simulink model "model_3"  (R2021b)
settings: Solver=VariableStepAuto  StartTime=0.0  StopTime=10  RelTol=1e-3
values from neighbouring files (symbols this model uses):
  A = [-5, 0; 0, -10]    [task_1.m]    (also in task_3.m = [0,1;0,0]; task_4.m = [0,1;0,0]; task_5.m = [0,1;0,0]; task_6.m = [0,1;0,0])
  B1 = [1,1;1,-1]    [task_3.m]    (also in task_4.m = [-2,1,0;-3,1,0]; task_5.m; task_6.m = [-2,1,0;-3,1,0])
  B2 = [0;1]    [task_3.m]    (also in task_4.m; task_5.m; task_6.m)
  C2 = [0,0;1,2;3,4]    [task_3.m]    (also in task_4.m = [1,2;3,0;0,0]; task_5.m = [0,0;2,3;]; task_6.m = [0,0;1,2])
  D2 = [5;0;0]    [task_3.m]    (also in task_4.m = [0;0;-2]; task_5.m = [1;0]; task_6.m = [-3; 0])
  K = -inv(D2'*D2)*B2'*Q    [task_3.m]    (also in task_4.m; task_5.m; task_6.m)
libraries: matrix_library x2
settings Model: Creator=vital  LastModifiedBy=vital

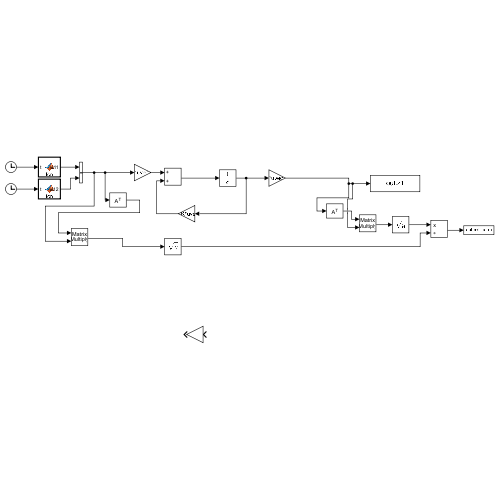
[thumbnail: Simulink's stored preview of the top-level diagram]
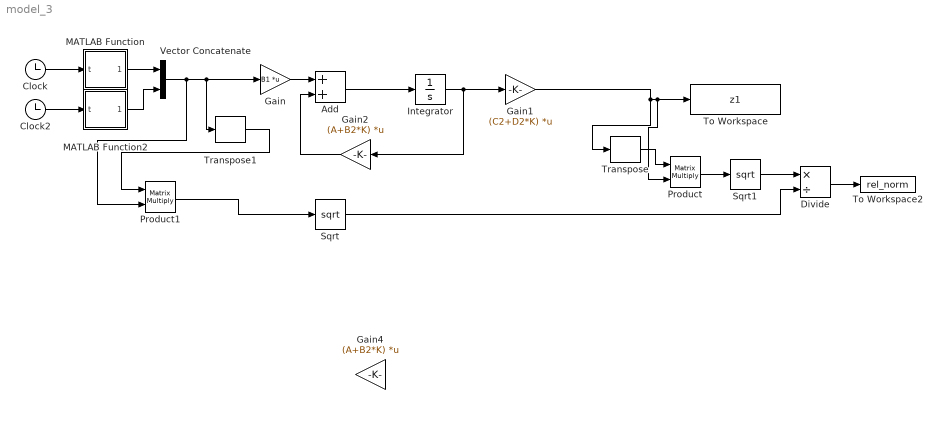
== system model_3 ==
  Add : Sum
  Clock : Clock
  Clock2 : Clock
  Divide : Product  Inputs=*/
  Gain : Gain  Gain=B1  Multiplication=Matrix(K*u) (u vector)
  Gain1 : Gain  Gain=(C2+D2*K)  Multiplication=Matrix(K*u) (u vector)
  Gain2 : Gain  Gain=(A+B2*K)  Multiplication=Matrix(K*u) (u vector)
  Gain4 : Gain  Gain=(A+B2*K)  Multiplication=Matrix(K*u) (u vector)
  Integrator : Integrator
  MATLAB Function : MATLAB Function  TreatAsAtomicUnit=on
  MATLAB Function2 : MATLAB Function  TreatAsAtomicUnit=on
  Product : Product  Multiplication=Matrix(*)
  Product1 : Product  Multiplication=Matrix(*)
  Sqrt : Sqrt  SaturateOnIntegerOverflow=on
  Sqrt1 : Sqrt  SaturateOnIntegerOverflow=on
  To Workspace : ToWorkspace  VariableName=z1  SaveFormat=Timeseries  SampleTime=0.0001
  To Workspace2 : ToWorkspace  VariableName=rel_norm  SaveFormat=Timeseries  SampleTime=0.0001
  Transpose : matrix_library/Transpose
      settings: SourceProductBaseCode=SL
  Transpose1 : matrix_library/Transpose
      settings: SourceProductBaseCode=SL
  Vector Concatenate : Concatenate
  wires:
  Integrator/1 -> Gain2/1, Gain1/1
  Transpose/1 -> Product/1
  Clock/1 -> MATLAB Function/1(t)
  Transpose1/1 -> Product1/1
  Product1/1 -> Sqrt/1
  Divide/1 -> To Workspace2/1
  Clock2/1 -> MATLAB Function2/1(t)
  MATLAB Function/1(w11) -> Vector Concatenate/1
  MATLAB Function2/1(w12) -> Vector Concatenate/2
  Vector Concatenate/1 -> Product1/2, Gain/1, Transpose1/1
  Sqrt/1 -> Divide/2
  Sqrt1/1 -> Divide/1
  Product/1 -> Sqrt1/1
  Gain/1 -> Add/1
  Add/1 -> Integrator/1
  Gain1/1 -> Product/2, To Workspace/1, Transpose/1
  Gain2/1 -> Add/2

== matlab function model_3/MATLAB Function2 ==
  data: t input; w12 output
function w12 = fcn(t)

w12 = 2*sin(t+pi/6);

== matlab function model_3/MATLAB Function ==
  data: t input; w11 output
function w11 = fcn(t)

w11 = sin(t);
